simulink model "kr_billiards_exam"  (R2017b)
settings: Solver=VariableStepAuto  StartTime=0.0  StopTime=40  RelTol=1e-3  EnableMultiTasking=on
PreLoadFcn:
  | addpath('Bill_Tables_STEP')
  | addpath('Skins')
  | addpath('Utilities')
  | addpath('Kuka_KR10_R1100_STEP')
model workspace (MATLAB code in the model file):
  | den=1.613292710828678e+03;
  | st=0.004;
  | Damping=0.2;
  | 
  | % Length of brick solid
  | L = 20; % cm
  | % Width of brick solid
  | W = 2; % cm
  | % Height of brick solid
  | H = 2; % cm
  | % Density of brick solid
  | rho = 1000; % kg/m^3
undefined symbols (not defined in the file or in its folder): ball_col, ball_x, ball_y, X, Y, Z
libraries: sm_lib x83, nesl_utility x64, fl_lib x12, simulink x5
(part 1 of 4)
settings Model: Creator=User  LastModifiedBy=Boris S. Notkin
settings DataIOCC: LimitDataPoints=on  SaveOutput=off  SignalLogging=off  DSMLogging=off  SaveTime=off
settings OptimizationCC: LifeSpan=inf
settings DebuggingCC: AllowSymbolicDim=off  SFUnexpectedBacktrackingDiag=warning  SFNoUnconditionalDefaultTransitionDiag=warning  SFExecutionAtInitializationDiag=none
settings CodeAppCC: StateflowObjectComments=on
settings GRTTargetCC: TargetLangStandard=C89/C90 (ANSI)  GeneratePreprocessorConditionals=Disable all
settings ConfigComp: CovMetricSettings=dw  CovHtmlReporting=on  CovSaveCumulativeToWorkspaceVar=on  CovSaveSingleToWorkspaceVar=on  CovExternalEMLEnable=off  CovSFcnEnable=off
settings SimscapeCC: SimscapeNominalValues="[{\"value\":\"10\",\"unit\":\"V\"},{\"value\":\"1\",\"unit\":\"A\"},{\"value\":\"10\",\"unit\":\"N*m\"},{\"value\":\"10\",\"unit\":\"bar\"},{\"value\":\"100\",\"unit\":\"kJ/kg\"},{\"value\":\"1\",\"unit\":\"kW\"},{\"value\":\"300\",\"unit\":\"K\"},{\"value\":\"100\",\"unit\":\"cm^3/s\"},{\"value\":\"1\",\"unit\":\"kN\"},{\"value\":\"1\",\"unit\":\"g/cm^3\"},{\"value\":\"1\",\"unit\":\"l\"},{\"value\":\"1\",\"unit\":\"cm^2\"},{\"value\":\"60\",\"unit\":\"Hz\"}]"  SimscapeLogDataHistory=10000
settings ExplorerConfigSet: InternalSimMechanicsExplorerSettings="<ExplorerConfiguration><canonicalview>default</canonicalview><AnimationSetting><BasePlaybackSpeed>1.0</BasePlaybackSpeed><PlaybackSpeedFactor>1.0</PlaybackSpeedFactor></AnimationSetting><TilePanel><TileInfo><Tiles Columns=\"1\" Count=\"1\" Rows=\"1\"><Column Weight=\"1\"/><Row Weight=\"1\"/><Tile Height=\"1\" Width=\"1\" X=\"0\" Y=\"0\"/></Tiles></TileInfo><SceneInfo><SceneViewer><BGColor><R>0.60000002384185791</R><G>0.60000002384185791</G><B>0.60000002384185791</B></BGColor><Camera><DoPerspective>off</DoPerspective><Position><X>2.11392585240804332</X><Y>-1.25242729688440968</Y><Z>1.30776618684503054</Z></Position><Center><X>0.66802137799346617</X><Y>0.19347717753016791</Y><Z>-0.138138287569547241</Z></Center><Up><X>-0.408248290463863073</X><Y>0.408248290463863073</Y><Z>0.816496580927726145</Z></Up><ViewLimDist>1</ViewLimDist><YLim>0.89923064778922468</YLim><XLim>1.35470687907166232</XLim></Camera></SceneViewer></SceneInfo></TilePanel><MechEditorPanel><Cameras><Camera><Id>Camera1</Id><Value><Name>Robot Camera</Name><NativeCamera><PositionTrackingFeature>Kuka_KR10.Axis7_R</PositionTrackingFeature><CenterTrackingFeature/><UpVectorTrackingFeature/><CenterTrackingOrigin>off</CenterTrackingOrigin><CenterTrackingDirection>+Z</CenterTrackingDirection><UpVectorTrackingDirection>-X</UpVectorTrackingDirection></NativeCamera></Value></Camera></Cameras><GfxPanelCameraMap/><VideoCreator><PlaybackSpeedRatio>1.0</PlaybackSpeedRatio><FrameRate>30</FrameRate><VideoFormat>Motion JPEG AVI</VideoFormat><FrameSize>auto</FrameSize></VideoCreator></MechEditorPanel></ExplorerConfiguration>"

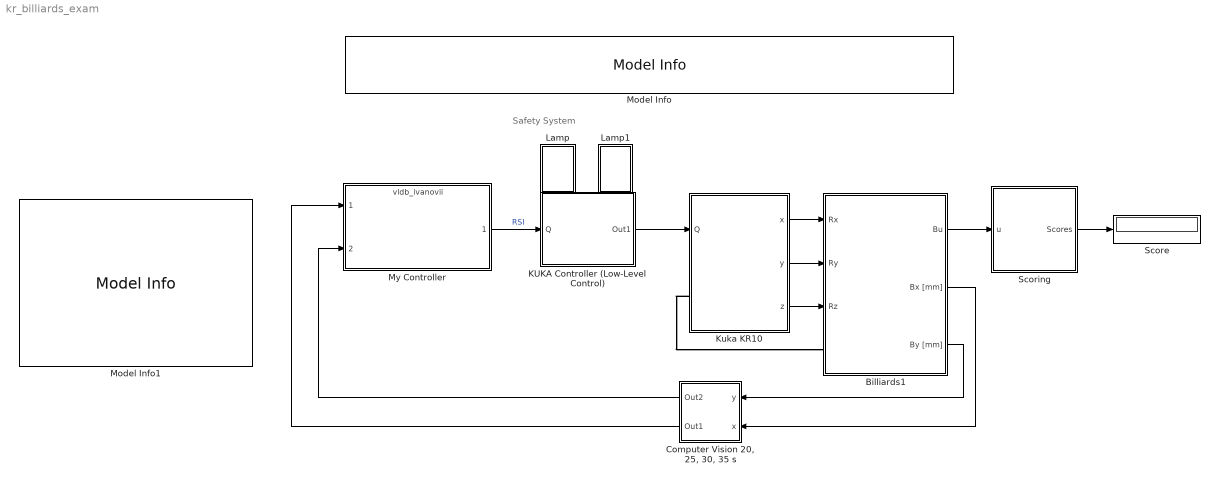
== system kr_billiards_exam ==
  note: Safety System
  Billiards1 : Subsystem
      mask init:
      | % [ball_x, ball_y, ball_col] = ball_and_cam_init_allocation(ball_mode, ball_rndfix, ...
      | %     ball_seed, foto_mode, foto_rndfix, foto_seed);
      mask DialogControl DescGroupVar Prompt: Размещение шаров на бильярдном столе и схема перемещения фотокамеры
      mask DialogControl DescTextVar Prompt: Выбор схемы размещения шаров на бильярдном шаре и схемы его обхода роботом, несущим фотокамеру системы компьютерного зрения.
      mask Display: image('billiard.jpg');
  "Computer Vision 20, 25, 30, 35 s" : Subsystem
      mask Display: image('comp_vis.jpg');
  KUKA Controller (Low-Level Control) : Subsystem  mask{min1=-170, max1=170, min2=-190, max2=45, min3=-120, max3=156, min4=-185, max4=185, min5=-120, max5=120, min6=-350, max6=350, EnableKinLim=on, acc1=600, acc2=450, acc3=450, acc4=762, acc5=622, acc6=984, EnableDynLim=on}
      mask prompts: min1 "Ось 1:"; min2 "Ось 2:"; min3 "Ось 3:"; min4 "Ось 4:"; min5 "Ось 5:"; min6 "Ось 6:"; EnableKinLim "Останавливать симуляцию при выходе за ограничения"; acc1 "Ось 1:"; acc2 "Ось 2:"; acc3 "Ось 3:"; acc4 "Ось 4:"; acc5 "Ось 5:"; acc6 "Ось 6:"; EnableDynLim "Останавливать симуляцию при выходе за ограничения"
      mask Callback EnableKinLim:
      | vis={'on','on','on','on','on','on','on','on','on','on','on','on','on','on','on','on','on','on','on','on'};
      | if strcmp(get_param(gcb,'EnableKinLim'),'off')
      |     for i=1:12
      |         vis{i}='off';
      |     end
      | end
      | if strcmp(get_param(gcb,'EnableDynLim'),'off')
      |     for i=14:19
      |         vis{i}='off';
      |     end
      | end
      | set_param(gcb,'MaskEnables',vis)
      mask Callback EnableDynLim:
      | vis={'on','on','on','on','on','on','on','on','on','on','on','on','on','on','on','on','on','on','on','on'};
      | if strcmp(get_param(gcb,'EnableKinLim'),'off')
      |     for i=1:12
      |         vis{i}='off';
      |     end
      | end
      | if strcmp(get_param(gcb,'EnableDynLim'),'off')
      |     for i=14:19
      |         vis{i}='off';
      |     end
      | end
      | set_param(gcb,'MaskEnables',vis)
      mask DialogControl ParameterGroupVar Prompt: Кинематические ограничения, град
      mask DialogControl Container3 Prompt: Динамические ограничения, град/c^2
      mask Display:
      | image('KR_C4.jpg');
      | port_label('input', 1, 'RSI')
  Kuka KR10 : Subsystem
      mask Display: image('kuka_kr10_r1100.jpg');
  Lamp : Subsystem  DialogController=hmiCreateDDGDialog  IsWebBlock=on  mask(MWDashboardBlock){webBlockId=50f85813-49c3-43b3-bc1d-ae04d07702bf, webBlockType=lamp, ShowInLibBrowser=on, ShowInitialText=on, HMISrcModelName=kr_billiards_exam}
      mask prompts: webBlockType "WebBlock Type"; HMISrcModelName "Source Model"
      mask help: SimulinkHMI:dialogs:LampDialogDesc
      mask Help: helpview([docroot '/mapfiles/simulink.map'], 'hmi_lamp')
      mask Display:
      | if strcmp(get_param(bdroot(gcb),'BlockDiagramType'), 'library')
      |     image([(matlabroot) '/toolbox/simulink/hmi/icons/Lamp.png']);
      | end
  Lamp1 : Subsystem  DialogController=hmiCreateDDGDialog  IsWebBlock=on  mask(MWDashboardBlock){webBlockId=c451b107-4d97-4e78-bf4d-8fc7e34e44b4, webBlockType=lamp, ShowInLibBrowser=on, ShowInitialText=on, HMISrcModelName=kr_billiards_exam}
      mask prompts: webBlockType "WebBlock Type"; HMISrcModelName "Source Model"
      mask help: SimulinkHMI:dialogs:LampDialogDesc
      mask Help: helpview([docroot '/mapfiles/simulink.map'], 'hmi_lamp')
      mask Display:
      | if strcmp(get_param(bdroot(gcb),'BlockDiagramType'), 'library')
      |     image([(matlabroot) '/toolbox/simulink/hmi/icons/Lamp.png']);
      | end
  Model Info : simulink/Model-Wide Utilities/Model Info  Frame=on  DisplayStringWithTags=Для запуска модели используйте скрипт EXAMINATOR.m  HorizontalTextAlignment=Center  LeftAlignmentValue=0.5
  Model Info1 : simulink/Model-Wide Utilities/Model Info  Frame=on  DisplayStringWithTags=|  HorizontalTextAlignment=Left  LeftAlignmentValue=0.02
      | Откройте на схеме блок My Controller (откроется 
      | модель участника) и в разделе описания модели
      | 
      | File/Model Properties//Model Properties/Description
      | 
      | укажите идентификационные данные участника 
      | Олимпиады.
      | 
      | 
      | Пример:
      | 
      | ФИО: Иванов Иван Иванович
      | ID: 123456789
      | Дата рождения: 23.02.1997
      | Email: ivanov@yandex.ru
      | Курс: Бакалавриат 4 курс
  My Controller : ModelReference  ModelNameDialog=vldb_ivanovii.slx  SimulationMode=Normal  ModelReferenceVersion=1.381
  Score : Display
  Scoring : Subsystem
      mask Display: image('scoring.jpg');
  wires:
  Kuka KR10/1(x) -> Billiards1/1(Rx)
  Kuka KR10/3(z) -> Billiards1/3(Rz)
  Kuka KR10/2(y) -> Billiards1/2(Ry)
  Billiards1/1(Bu) -> Scoring/1(u)
  Scoring/1(Scores) -> Score/1
  KUKA Controller (Low-Level Control)/1(Out1) -> Kuka KR10/1(Q)
  Billiards1/2(Bx [mm]) -> "Computer Vision 20, 25, 30, 35 s"/2(x)
  Billiards1/3(By [mm]) -> "Computer Vision 20, 25, 30, 35 s"/1(y)
  "Computer Vision 20, 25, 30, 35 s"/1(Out2) -> My Controller/2
  "Computer Vision 20, 25, 30, 35 s"/2(Out1) -> My Controller/1
  My Controller/1 -> KUKA Controller (Low-Level Control)/1(Q)  "RSI"
  connections:
  Kuka KR10/LConn1 -- Billiards1/LConn1

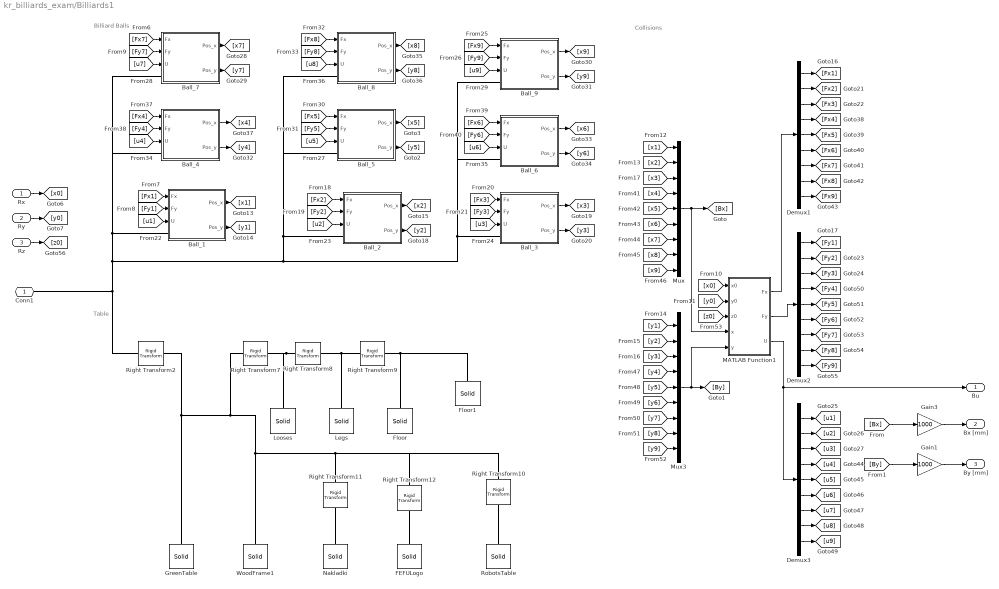
== system kr_billiards_exam/Billiards1 ==
  note: Collisions
  note: Billiard Balls
  note: Table
  Rx : Inport
  Ry : Inport  Port=2
  Rz : Inport  Port=3
  Ball_1 : Subsystem  mask{x0=ball_x(1), y0=ball_y(1), d=Damping, pd=5, rgb=ball_col(1,:)}
      mask prompts: d "Damping"; pd "Parking damping"; rgb "Color"
  Ball_2 : Subsystem  mask{x0=ball_x(2), y0=ball_y(2), d=Damping, pd=5, rgb=ball_col(2,:)}
      mask prompts: d "Damping"; pd "Parking damping"; rgb "Color"
  Ball_3 : Subsystem  mask{x0=ball_x(3), y0=ball_y(3), d=Damping, pd=5, rgb=ball_col(3,:)}
      mask prompts: d "Damping"; pd "Parking damping"; rgb "Color"
  Ball_4 : Subsystem  mask{x0=ball_x(4), y0=ball_y(4), d=Damping, pd=5, rgb=ball_col(4,:)}
      mask prompts: d "Damping"; pd "Parking damping"; rgb "Color"
  Ball_5 : Subsystem  mask{x0=ball_x(5), y0=ball_y(5), d=Damping, pd=5, rgb=ball_col(5,:)}
      mask prompts: d "Damping"; pd "Parking damping"; rgb "Color"
  Ball_6 : Subsystem  mask{x0=ball_x(6), y0=ball_y(6), d=Damping, pd=5, rgb=ball_col(6,:)}
      mask prompts: d "Damping"; pd "Parking damping"; rgb "Color"
  Ball_7 : Subsystem  mask{x0=ball_x(7), y0=ball_y(7), d=Damping, pd=5, rgb=ball_col(7,:)}
      mask prompts: d "Damping"; pd "Parking damping"; rgb "Color"
  Ball_8 : Subsystem  mask{x0=ball_x(8), y0=ball_y(8), d=Damping, pd=5, rgb=ball_col(8,:)}
      mask prompts: d "Damping"; pd "Parking damping"; rgb "Color"
  Ball_9 : Subsystem  mask{x0=ball_x(9), y0=ball_y(9), d=Damping, pd=5, rgb=ball_col(9,:)}
      mask prompts: d "Damping"; pd "Parking damping"; rgb "Color"
  Demux1 : Demux  Outputs=9
  Demux2 : Demux  Outputs=9
  Demux3 : Demux  Outputs=9
  FEFULogo : sm_lib/Body Elements/Solid  InertiaType=CalculateFromGeometry  Mass=1  MassUnits=kg  CenterOfMass=[0 0 0]  CenterOfMassUnits=m  MomentsOfInertia=[1 1 1]  MomentsOfInertiaUnits=kg*m^2  ProductsOfInertia=[0 0 0]  ProductsOfInertiaUnits=kg*m^2  DensityBased=on  Density=rho  DensityUnits=kg/m^3  DoExposeReferenceFrame=on  SerializedFrames=<Frames/>  GraphicType=FromGeometry  MarkerShape=Sphere  MarkerSize=1  MarkerSizeUnits=m  GraphicVisPropType=SimpleVisualProperties  GraphicDiffuseColor=[1.0 0.8 0.0]  GraphicSpecularColor=[0.2 0.2 0.2]  GraphicAmbientColor=[0.5 0.5 0.5]  GraphicEmissiveColor=[0.1 0.1 0.1]  GraphicShininess=24.0  GraphicOpacity=1  GeometryShape=FromFile  RectangleSize=[1 1]  RectangleSizeUnits=m  BrickDimensions=[L W H]  BrickDimensionUnits=cm  CylinderRadius=1  CylinderRadiusUnits=m  CylinderLength=1  CylinderLengthUnits=m  SphereRadius=1  SphereRadiusUnits=m  EllipsoidRadii=[1 1 1]  EllipsoidRadiiUnits=m  ExtrusionCrossSection=[1 1; -1 1; -1 -1; 1 -1]  ExtrusionCrossSectionUnits=m  ExtrusionLength=1  ExtrusionLengthUnits=m  PolygonNumSides=1  PolygonOuterRadius=1  PolygonOuterRadiusUnits=m  ExtGeomFileType=STEP  ExtGeomFileName=FEFULogo.STEP  ExtGeomFileUnits=m  RevolutionCrossSection=[1 1; 1 -1; 2 -1; 2 1]  RevolutionCrossSectionUnits=m  RevolutionExtent=Full  RevolutionAngle=180  RevolutionAngleUnits=deg
  Floor : sm_lib/Body Elements/Solid  InertiaType=CalculateFromGeometry  Mass=1  MassUnits=kg  CenterOfMass=[0 0 0]  CenterOfMassUnits=m  MomentsOfInertia=[1 1 1]  MomentsOfInertiaUnits=kg*m^2  ProductsOfInertia=[0 0 0]  ProductsOfInertiaUnits=kg*m^2  DensityBased=on  Density=rho  DensityUnits=kg/m^3  DoExposeReferenceFrame=on  SerializedFrames=<Frames/>  GraphicType=FromGeometry  MarkerShape=Sphere  MarkerSize=1  MarkerSizeUnits=m  GraphicVisPropType=SimpleVisualProperties  GraphicDiffuseColor=[1.0 1.0 1.0]  GraphicSpecularColor=[0.2 0.2 0.2]  GraphicAmbientColor=[0.5 0.5 0.5]  GraphicEmissiveColor=[0.1 0.1 0.1]  GraphicShininess=24.0  GraphicOpacity=1  GeometryShape=FromFile  RectangleSize=[1 1]  RectangleSizeUnits=m  BrickDimensions=[L W H]  BrickDimensionUnits=cm  CylinderRadius=1  CylinderRadiusUnits=m  CylinderLength=1  CylinderLengthUnits=m  SphereRadius=1  SphereRadiusUnits=m  EllipsoidRadii=[1 1 1]  EllipsoidRadiiUnits=m  ExtrusionCrossSection=[1 1; -1 1; -1 -1; 1 -1]  ExtrusionCrossSectionUnits=m  ExtrusionLength=1  ExtrusionLengthUnits=m  PolygonNumSides=1  PolygonOuterRadius=1  PolygonOuterRadiusUnits=m  ExtGeomFileType=STEP  ExtGeomFileName=Floor.STEP  ExtGeomFileUnits=m  RevolutionCrossSection=[1 1; 1 -1; 2 -1; 2 1]  RevolutionCrossSectionUnits=m  RevolutionExtent=Full  RevolutionAngle=180  RevolutionAngleUnits=deg
  Floor1 : sm_lib/Body Elements/Solid  InertiaType=CalculateFromGeometry  Mass=1  MassUnits=kg  CenterOfMass=[0 0 0]  CenterOfMassUnits=m  MomentsOfInertia=[1 1 1]  MomentsOfInertiaUnits=kg*m^2  ProductsOfInertia=[0 0 0]  ProductsOfInertiaUnits=kg*m^2  DensityBased=on  Density=rho  DensityUnits=kg/m^3  DoExposeReferenceFrame=on  SerializedFrames=<Frames/>  GraphicType=FromGeometry  MarkerShape=Sphere  MarkerSize=1  MarkerSizeUnits=m  GraphicVisPropType=SimpleVisualProperties  GraphicDiffuseColor=[0.3 0.3 0.3]  GraphicSpecularColor=[0.2 0.2 0.2]  GraphicAmbientColor=[0.5 0.5 0.5]  GraphicEmissiveColor=[0.1 0.1 0.1]  GraphicShininess=24.0  GraphicOpacity=1  GeometryShape=Brick  RectangleSize=[1 1]  RectangleSizeUnits=m  BrickDimensions=[6 3 0.003]  BrickDimensionUnits=m  CylinderRadius=1  CylinderRadiusUnits=m  CylinderLength=1  CylinderLengthUnits=m  SphereRadius=1  SphereRadiusUnits=m  EllipsoidRadii=[1 1 1]  EllipsoidRadiiUnits=m  ExtrusionCrossSection=[1 1; -1 1; -1 -1; 1 -1]  ExtrusionCrossSectionUnits=m  ExtrusionLength=1  ExtrusionLengthUnits=m  PolygonNumSides=1  PolygonOuterRadius=1  PolygonOuterRadiusUnits=m  ExtGeomFileType=STEP  ExtGeomFileName=C:\PingPong\BillTablesSTEPDecor2\Floor.STEP  ExtGeomFileUnits=m  RevolutionCrossSection=[1 1; 1 -1; 2 -1; 2 1]  RevolutionCrossSectionUnits=m  RevolutionExtent=Full  RevolutionAngle=180  RevolutionAngleUnits=deg
  Gain1 : Gain  Gain=1000
  Gain3 : Gain  Gain=1000
  GreenTable : sm_lib/Body Elements/Solid  InertiaType=CalculateFromGeometry  Mass=1  MassUnits=kg  CenterOfMass=[0 0 0]  CenterOfMassUnits=m  MomentsOfInertia=[1 1 1]  MomentsOfInertiaUnits=kg*m^2  ProductsOfInertia=[0 0 0]  ProductsOfInertiaUnits=kg*m^2  DensityBased=on  Density=rho  DensityUnits=kg/m^3  DoExposeReferenceFrame=on  SerializedFrames=<Frames/>  GraphicType=FromGeometry  MarkerShape=Sphere  MarkerSize=1  MarkerSizeUnits=m  GraphicVisPropType=SimpleVisualProperties  GraphicDiffuseColor=[0.0 0.8 0.2]  GraphicSpecularColor=[0.2 0.2 0.2]  GraphicAmbientColor=[0.5 0.5 0.5]  GraphicEmissiveColor=[0.1 0.1 0.1]  GraphicShininess=24.0  GraphicOpacity=1  GeometryShape=FromFile  RectangleSize=[1 1]  RectangleSizeUnits=m  BrickDimensions=[L W H]  BrickDimensionUnits=cm  CylinderRadius=1  CylinderRadiusUnits=m  CylinderLength=1  CylinderLengthUnits=m  SphereRadius=1  SphereRadiusUnits=m  EllipsoidRadii=[1 1 1]  EllipsoidRadiiUnits=m  ExtrusionCrossSection=[1 1; -1 1; -1 -1; 1 -1]  ExtrusionCrossSectionUnits=m  ExtrusionLength=1  ExtrusionLengthUnits=m  PolygonNumSides=1  PolygonOuterRadius=1  PolygonOuterRadiusUnits=m  ExtGeomFileType=STEP  ExtGeomFileName=GreenTable.STEP  ExtGeomFileUnits=m  RevolutionCrossSection=[1 1; 1 -1; 2 -1; 2 1]  RevolutionCrossSectionUnits=m  RevolutionExtent=Full  RevolutionAngle=180  RevolutionAngleUnits=deg
  Legs : sm_lib/Body Elements/Solid  InertiaType=CalculateFromGeometry  Mass=1  MassUnits=kg  CenterOfMass=[0 0 0]  CenterOfMassUnits=m  MomentsOfInertia=[1 1 1]  MomentsOfInertiaUnits=kg*m^2  ProductsOfInertia=[0 0 0]  ProductsOfInertiaUnits=kg*m^2  DensityBased=on  Density=rho  DensityUnits=kg/m^3  DoExposeReferenceFrame=on  SerializedFrames=<Frames/>  GraphicType=FromGeometry  MarkerShape=Sphere  MarkerSize=1  MarkerSizeUnits=m  GraphicVisPropType=SimpleVisualProperties  GraphicDiffuseColor=[1.0 0.8 0.4]  GraphicSpecularColor=[0.2 0.2 0.2]  GraphicAmbientColor=[0.5 0.5 0.5]  GraphicEmissiveColor=[0.1 0.1 0.1]  GraphicShininess=24.0  GraphicOpacity=1  GeometryShape=FromFile  RectangleSize=[1 1]  RectangleSizeUnits=m  BrickDimensions=[L W H]  BrickDimensionUnits=cm  CylinderRadius=1  CylinderRadiusUnits=m  CylinderLength=1  CylinderLengthUnits=m  SphereRadius=1  SphereRadiusUnits=m  EllipsoidRadii=[1 1 1]  EllipsoidRadiiUnits=m  ExtrusionCrossSection=[1 1; -1 1; -1 -1; 1 -1]  ExtrusionCrossSectionUnits=m  ExtrusionLength=1  ExtrusionLengthUnits=m  PolygonNumSides=1  PolygonOuterRadius=1  PolygonOuterRadiusUnits=m  ExtGeomFileType=STEP  ExtGeomFileName=Legs.STEP  ExtGeomFileUnits=m  RevolutionCrossSection=[1 1; 1 -1; 2 -1; 2 1]  RevolutionCrossSectionUnits=m  RevolutionExtent=Full  RevolutionAngle=180  RevolutionAngleUnits=deg
  Looses : sm_lib/Body Elements/Solid  InertiaType=CalculateFromGeometry  Mass=1  MassUnits=kg  CenterOfMass=[0 0 0]  CenterOfMassUnits=m  MomentsOfInertia=[1 1 1]  MomentsOfInertiaUnits=kg*m^2  ProductsOfInertia=[0 0 0]  ProductsOfInertiaUnits=kg*m^2  DensityBased=on  Density=rho  DensityUnits=kg/m^3  DoExposeReferenceFrame=on  SerializedFrames=<Frames/>  GraphicType=FromGeometry  MarkerShape=Sphere  MarkerSize=1  MarkerSizeUnits=m  GraphicVisPropType=SimpleVisualProperties  GraphicDiffuseColor=[0.2 0.2 0.2]  GraphicSpecularColor=[0.2 0.2 0.2]  GraphicAmbientColor=[0.5 0.5 0.5]  GraphicEmissiveColor=[0.1 0.1 0.1]  GraphicShininess=24.0  GraphicOpacity=1  GeometryShape=FromFile  RectangleSize=[1 1]  RectangleSizeUnits=m  BrickDimensions=[L W H]  BrickDimensionUnits=cm  CylinderRadius=1  CylinderRadiusUnits=m  CylinderLength=1  CylinderLengthUnits=m  SphereRadius=1  SphereRadiusUnits=m  EllipsoidRadii=[1 1 1]  EllipsoidRadiiUnits=m  ExtrusionCrossSection=[1 1; -1 1; -1 -1; 1 -1]  ExtrusionCrossSectionUnits=m  ExtrusionLength=1  ExtrusionLengthUnits=m  PolygonNumSides=1  PolygonOuterRadius=1  PolygonOuterRadiusUnits=m  ExtGeomFileType=STEP  ExtGeomFileName=Looses.STEP  ExtGeomFileUnits=m  RevolutionCrossSection=[1 1; 1 -1; 2 -1; 2 1]  RevolutionCrossSectionUnits=m  RevolutionExtent=Full  RevolutionAngle=180  RevolutionAngleUnits=deg
  MATLAB Function1 : MATLAB Function  TreatAsAtomicUnit=on
  Mux : Mux  Inputs=9
  Mux3 : Mux  Inputs=9
  Nakladki : sm_lib/Body Elements/Solid  InertiaType=CalculateFromGeometry  Mass=1  MassUnits=kg  CenterOfMass=[0 0 0]  CenterOfMassUnits=m  MomentsOfInertia=[1 1 1]  MomentsOfInertiaUnits=kg*m^2  ProductsOfInertia=[0 0 0]  ProductsOfInertiaUnits=kg*m^2  DensityBased=on  Density=rho  DensityUnits=kg/m^3  DoExposeReferenceFrame=on  SerializedFrames=<Frames/>  GraphicType=FromGeometry  MarkerShape=Sphere  MarkerSize=1  MarkerSizeUnits=m  GraphicVisPropType=SimpleVisualProperties  GraphicDiffuseColor=[1.0 0.8 0.0]  GraphicSpecularColor=[0.2 0.2 0.2]  GraphicAmbientColor=[0.5 0.5 0.5]  GraphicEmissiveColor=[0.1 0.1 0.1]  GraphicShininess=24.0  GraphicOpacity=1  GeometryShape=FromFile  RectangleSize=[1 1]  RectangleSizeUnits=m  BrickDimensions=[L W H]  BrickDimensionUnits=cm  CylinderRadius=1  CylinderRadiusUnits=m  CylinderLength=1  CylinderLengthUnits=m  SphereRadius=1  SphereRadiusUnits=m  EllipsoidRadii=[1 1 1]  EllipsoidRadiiUnits=m  ExtrusionCrossSection=[1 1; -1 1; -1 -1; 1 -1]  ExtrusionCrossSectionUnits=m  ExtrusionLength=1  ExtrusionLengthUnits=m  PolygonNumSides=1  PolygonOuterRadius=1  PolygonOuterRadiusUnits=m  ExtGeomFileType=STEP  ExtGeomFileName=Nakladki.STEP  ExtGeomFileUnits=m  RevolutionCrossSection=[1 1; 1 -1; 2 -1; 2 1]  RevolutionCrossSectionUnits=m  RevolutionExtent=Full  RevolutionAngle=180  RevolutionAngleUnits=deg
  Right Transform10 : sm_lib/Frames and Transforms/Rigid Transform  TranslationMethod=Cartesian  TranslationStandardOffset=L/2  TranslationLengthUnit=mm  TranslationStandardAxis=+X  TranslationCartesianOffset=[0 0 -523.67]  TranslationROffset=0  TranslationROffsetUnits=m  TranslationZOffset=0  TranslationZOffsetUnits=m  TranslationThetaOffset=0  TranslationThetaOffsetUnits=deg  RotationMethod=AlignedAxes  RotationAngleUnits=deg  RotationStandardAxis=+Z  RotationAngle=0  RotationArbitraryAxis=[0 0 1]  FollAlignAxisA=+Z  BaseAlignAxisA=+Z  FollAlignAxisB=+X  BaseAlignAxisB=+X  RotationSequenceAxes=FollowerAxes  RotationSequence=XYX  RotationSequenceAngles=[0 0 0]  RotationSequenceAnglesUnits=deg  RotationMatrix=[1 0 0; 0 1 0; 0 0 1]
  Right Transform11 : sm_lib/Frames and Transforms/Rigid Transform  TranslationMethod=Cartesian  TranslationStandardOffset=L/2  TranslationLengthUnit=mm  TranslationStandardAxis=+X  TranslationCartesianOffset=[0 50 0]  TranslationROffset=0  TranslationROffsetUnits=m  TranslationZOffset=0  TranslationZOffsetUnits=m  TranslationThetaOffset=0  TranslationThetaOffsetUnits=deg  RotationMethod=AlignedAxes  RotationAngleUnits=deg  RotationStandardAxis=+Z  RotationAngle=0  RotationArbitraryAxis=[0 0 1]  FollAlignAxisA=+Z  BaseAlignAxisA=+Y  FollAlignAxisB=+Y  BaseAlignAxisB=+Z  RotationSequenceAxes=FollowerAxes  RotationSequence=XYX  RotationSequenceAngles=[0 0 0]  RotationSequenceAnglesUnits=deg  RotationMatrix=[1 0 0; 0 1 0; 0 0 1]
  Right Transform12 : sm_lib/Frames and Transforms/Rigid Transform  TranslationMethod=Cartesian  TranslationStandardOffset=L/2  TranslationLengthUnit=mm  TranslationStandardAxis=+X  TranslationCartesianOffset=[0 -460.09 0]  TranslationROffset=0  TranslationROffsetUnits=m  TranslationZOffset=0  TranslationZOffsetUnits=m  TranslationThetaOffset=0  TranslationThetaOffsetUnits=deg  RotationMethod=AlignedAxes  RotationAngleUnits=deg  RotationStandardAxis=+Z  RotationAngle=0  RotationArbitraryAxis=[0 0 1]  FollAlignAxisA=+Z  BaseAlignAxisA=+Z  FollAlignAxisB=+X  BaseAlignAxisB=+X  RotationSequenceAxes=FollowerAxes  RotationSequence=XYX  RotationSequenceAngles=[0 0 0]  RotationSequenceAnglesUnits=deg  RotationMatrix=[1 0 0; 0 1 0; 0 0 1]
  Right Transform2 : sm_lib/Frames and Transforms/Rigid Transform  TranslationMethod=Cartesian  TranslationStandardOffset=L/2  TranslationLengthUnit=mm  TranslationStandardAxis=+X  TranslationCartesianOffset=[725 0 70]  TranslationROffset=0  TranslationROffsetUnits=m  TranslationZOffset=0  TranslationZOffsetUnits=m  TranslationThetaOffset=0  TranslationThetaOffsetUnits=deg  RotationMethod=RotationSequence  RotationAngleUnits=deg  RotationStandardAxis=+Z  RotationAngle=0  RotationArbitraryAxis=[0 0 1]  FollAlignAxisA=+X  BaseAlignAxisA=-Y  FollAlignAxisB=+Y  BaseAlignAxisB=-X  RotationSequenceAxes=FollowerAxes  RotationSequence=ZYX  RotationSequenceAngles=[90 0 90]  RotationSequenceAnglesUnits=deg  RotationMatrix=[1 0 0; 0 1 0; 0 0 1]
  Right Transform7 : sm_lib/Frames and Transforms/Rigid Transform  TranslationMethod=Cartesian  TranslationStandardOffset=L/2  TranslationLengthUnit=mm  TranslationStandardAxis=+X  TranslationCartesianOffset=[0 0 0]  TranslationROffset=0  TranslationROffsetUnits=m  TranslationZOffset=0  TranslationZOffsetUnits=m  TranslationThetaOffset=0  TranslationThetaOffsetUnits=deg  RotationMethod=AlignedAxes  RotationAngleUnits=deg  RotationStandardAxis=+Z  RotationAngle=0  RotationArbitraryAxis=[0 0 1]  FollAlignAxisA=+Z  BaseAlignAxisA=+Y  FollAlignAxisB=+Y  BaseAlignAxisB=+Z  RotationSequenceAxes=FollowerAxes  RotationSequence=XYX  RotationSequenceAngles=[0 0 0]  RotationSequenceAnglesUnits=deg  RotationMatrix=[1 0 0; 0 1 0; 0 0 1]
  Right Transform8 : sm_lib/Frames and Transforms/Rigid Transform  TranslationMethod=Cartesian  TranslationStandardOffset=L/2  TranslationLengthUnit=mm  TranslationStandardAxis=+X  TranslationCartesianOffset=[0 0 0]  TranslationROffset=0  TranslationROffsetUnits=m  TranslationZOffset=0  TranslationZOffsetUnits=m  TranslationThetaOffset=0  TranslationThetaOffsetUnits=deg  RotationMethod=AlignedAxes  RotationAngleUnits=deg  RotationStandardAxis=+Z  RotationAngle=0  RotationArbitraryAxis=[0 0 1]  FollAlignAxisA=+Z  BaseAlignAxisA=+Y  FollAlignAxisB=+Y  BaseAlignAxisB=+Z  RotationSequenceAxes=FollowerAxes  RotationSequence=XYX  RotationSequenceAngles=[0 0 0]  RotationSequenceAnglesUnits=deg  RotationMatrix=[1 0 0; 0 1 0; 0 0 1]
  Right Transform9 : sm_lib/Frames and Transforms/Rigid Transform  TranslationMethod=Cartesian  TranslationStandardOffset=L/2  TranslationLengthUnit=mm  TranslationStandardAxis=+X  TranslationCartesianOffset=[0 -461.09 0]  TranslationROffset=0  TranslationROffsetUnits=m  TranslationZOffset=0  TranslationZOffsetUnits=m  TranslationThetaOffset=0  TranslationThetaOffsetUnits=deg  RotationMethod=AlignedAxes  RotationAngleUnits=deg  RotationStandardAxis=+Z  RotationAngle=0  RotationArbitraryAxis=[0 0 1]  FollAlignAxisA=+Z  BaseAlignAxisA=+Y  FollAlignAxisB=+Y  BaseAlignAxisB=+Z  RotationSequenceAxes=FollowerAxes  RotationSequence=XYX  RotationSequenceAngles=[0 0 0]  RotationSequenceAnglesUnits=deg  RotationMatrix=[1 0 0; 0 1 0; 0 0 1]
  RobotsTable : sm_lib/Body Elements/Solid  InertiaType=CalculateFromGeometry  Mass=1  MassUnits=kg  CenterOfMass=[0 0 0]  CenterOfMassUnits=m  MomentsOfInertia=[1 1 1]  MomentsOfInertiaUnits=kg*m^2  ProductsOfInertia=[0 0 0]  ProductsOfInertiaUnits=kg*m^2  DensityBased=on  Density=rho  DensityUnits=kg/m^3  DoExposeReferenceFrame=on  SerializedFrames=<Frames/>  GraphicType=FromGeometry  MarkerShape=Sphere  MarkerSize=1  MarkerSizeUnits=m  GraphicVisPropType=SimpleVisualProperties  GraphicDiffuseColor=[0.4 0.4 0.4]  GraphicSpecularColor=[0.2 0.2 0.2]  GraphicAmbientColor=[0.5 0.5 0.5]  GraphicEmissiveColor=[0.1 0.1 0.1]  GraphicShininess=24.0  GraphicOpacity=1  GeometryShape=FromFile  RectangleSize=[1 1]  RectangleSizeUnits=m  BrickDimensions=[L W H]  BrickDimensionUnits=cm  CylinderRadius=1  CylinderRadiusUnits=m  CylinderLength=1  CylinderLengthUnits=m  SphereRadius=1  SphereRadiusUnits=m  EllipsoidRadii=[1 1 1]  EllipsoidRadiiUnits=m  ExtrusionCrossSection=[1 1; -1 1; -1 -1; 1 -1]  ExtrusionCrossSectionUnits=m  ExtrusionLength=1  ExtrusionLengthUnits=m  PolygonNumSides=1  PolygonOuterRadius=1  PolygonOuterRadiusUnits=m  ExtGeomFileType=STEP  ExtGeomFileName=RobotsTable.STEP  ExtGeomFileUnits=m  RevolutionCrossSection=[1 1; 1 -1; 2 -1; 2 1]  RevolutionCrossSectionUnits=m  RevolutionExtent=Full  RevolutionAngle=180  RevolutionAngleUnits=deg
  WoodFrame1 : sm_lib/Body Elements/Solid  InertiaType=CalculateFromGeometry  Mass=1  MassUnits=kg  CenterOfMass=[0 0 0]  CenterOfMassUnits=m  MomentsOfInertia=[1 1 1]  MomentsOfInertiaUnits=kg*m^2  ProductsOfInertia=[0 0 0]  ProductsOfInertiaUnits=kg*m^2  DensityBased=on  Density=rho  DensityUnits=kg/m^3  DoExposeReferenceFrame=on  SerializedFrames=<Frames/>  GraphicType=FromGeometry  MarkerShape=Sphere  MarkerSize=1  MarkerSizeUnits=m  GraphicVisPropType=SimpleVisualProperties  GraphicDiffuseColor=[1.0 0.4 0.0]  GraphicSpecularColor=[0.2 0.2 0.2]  GraphicAmbientColor=[0.5 0.5 0.5]  GraphicEmissiveColor=[0.1 0.1 0.1]  GraphicShininess=24.0  GraphicOpacity=1  GeometryShape=FromFile  RectangleSize=[1 1]  RectangleSizeUnits=m  BrickDimensions=[L W H]  BrickDimensionUnits=cm  CylinderRadius=1  CylinderRadiusUnits=m  CylinderLength=1  CylinderLengthUnits=m  SphereRadius=1  SphereRadiusUnits=m  EllipsoidRadii=[1 1 1]  EllipsoidRadiiUnits=m  ExtrusionCrossSection=[1 1; -1 1; -1 -1; 1 -1]  ExtrusionCrossSectionUnits=m  ExtrusionLength=1  ExtrusionLengthUnits=m  PolygonNumSides=1  PolygonOuterRadius=1  PolygonOuterRadiusUnits=m  ExtGeomFileType=STEP  ExtGeomFileName=WoodFrame.STEP  ExtGeomFileUnits=m  RevolutionCrossSection=[1 1; 1 -1; 2 -1; 2 1]  RevolutionCrossSectionUnits=m  RevolutionExtent=Full  RevolutionAngle=180  RevolutionAngleUnits=deg
  Conn1 : PMIOPort  Port=1  Side=Left
  Bu : Outport
  Bx [mm] : Outport  Port=2
  By [mm] : Outport  Port=3
  wires:
  [u5] -> Ball_5/3(U)
  Ball_9/2(Pos_y) -> [y9]
  [Fy4] -> Ball_4/2(Fy)
  [u7] -> Ball_7/3(U)
  [Fy8] -> Ball_8/2(Fy)
  [Fx8] -> Ball_8/1(Fx)
  [Fy3] -> Ball_3/2(Fy)
  Ball_8/2(Pos_y) -> [y8]
  [Fy6] -> Ball_6/2(Fy)
  [Fy2] -> Ball_2/2(Fy)
  [Fx4] -> Ball_4/1(Fx)
  Ball_1/2(Pos_y) -> [y1]
  Ball_1/1(Pos_x) -> [x1]
  [u2] -> Ball_2/3(U)
  Ball_5/1(Pos_x) -> [x5]
  [u4] -> Ball_4/3(U)
  [Fx3] -> Ball_3/1(Fx)
  [Fy9] -> Ball_9/2(Fy)
  Ball_5/2(Pos_y) -> [y5]
  Ball_2/2(Pos_y) -> [y2]
  Ball_9/1(Pos_x) -> [x9]
  Ball_4/1(Pos_x) -> [x4]
  Ball_3/1(Pos_x) -> [x3]
  [u6] -> Ball_6/3(U)
  Ball_2/1(Pos_x) -> [x2]
  Ball_8/1(Pos_x) -> [x8]
  [Fx1] -> Ball_1/1(Fx)
  Ball_6/1(Pos_x) -> [x6]
  Ball_3/2(Pos_y) -> [y3]
  [u1] -> Ball_1/3(U)
  [Fx6] -> Ball_6/1(Fx)
  [Fy1] -> Ball_1/2(Fy)
  [Fy7] -> Ball_7/2(Fy)
  [u9] -> Ball_9/3(U)
  [Fx2] -> Ball_2/1(Fx)
  [Fx5] -> Ball_5/1(Fx)
  Ball_6/2(Pos_y) -> [y6]
  Ball_7/1(Pos_x) -> [x7]
  Ball_4/2(Pos_y) -> [y4]
  [Fx9] -> Ball_9/1(Fx)
  [u3] -> Ball_3/3(U)
  [Fx7] -> Ball_7/1(Fx)
  Ball_7/2(Pos_y) -> [y7]
  [u8] -> Ball_8/3(U)
  [Fy5] -> Ball_5/2(Fy)
  Rz/1 -> [z0]
  Rx/1 -> [x0]
  Ry/1 -> [y0]
  MATLAB Function1/1(Fx) -> Demux1/1
  Mux/1 -> [Bx], MATLAB Function1/4(x)
  Mux3/1 -> [By], MATLAB Function1/5(y)
  MATLAB Function1/3(U) -> Demux3/1, Bu/1
  MATLAB Function1/2(Fy) -> Demux2/1
  [z0] -> MATLAB Function1/3(z0)
  [x0] -> MATLAB Function1/1(x0)
  [y0] -> MATLAB Function1/2(y0)
  [x1] -> Mux/1
  [x2] -> Mux/2
  [x3] -> Mux/3
  [x4] -> Mux/4
  [x5] -> Mux/5
  [x6] -> Mux/6
  [x7] -> Mux/7
  [x8] -> Mux/8
  [x9] -> Mux/9
  [y1] -> Mux3/1
  [y2] -> Mux3/2
  [y3] -> Mux3/3
  [y4] -> Mux3/4
  [y5] -> Mux3/5
  [y6] -> Mux3/6
  [y7] -> Mux3/7
  [y8] -> Mux3/8
  [y9] -> Mux3/9
  Demux1/1 -> [Fx1]
  Demux1/2 -> [Fx2]
  Demux1/3 -> [Fx3]
  Demux1/4 -> [Fx4]
  Demux1/5 -> [Fx5]
  Demux1/6 -> [Fx6]
  Demux1/7 -> [Fx7]
  Demux1/8 -> [Fx8]
  Demux1/9 -> [Fx9]
  Demux2/1 -> [Fy1]
  Demux2/2 -> [Fy2]
  Demux2/3 -> [Fy3]
  Demux2/4 -> [Fy4]
  Demux2/5 -> [Fy5]
  Demux2/6 -> [Fy6]
  Demux2/7 -> [Fy7]
  Demux2/8 -> [Fy8]
  Demux2/9 -> [Fy9]
  Demux3/1 -> [u1]
  Demux3/2 -> [u2]
  Demux3/3 -> [u3]
  Demux3/4 -> [u4]
  Demux3/5 -> [u5]
  Demux3/6 -> [u6]
  Demux3/7 -> [u7]
  Demux3/8 -> [u8]
  Demux3/9 -> [u9]
  [Bx] -> Gain3/1
  [By] -> Gain1/1
  Gain3/1 -> Bx [mm]/1
  Gain1/1 -> By [mm]/1
  connections:
  Conn1/RConn1 -- Ball_7/LConn1 -- Ball_4/LConn1 -- Ball_1/LConn1 -- Ball_8/LConn1 -- Ball_5/LConn1 -- Ball_2/LConn1 -- Ball_9/LConn1 -- Ball_6/LConn1 -- Ball_3/LConn1 -- Right Transform2/LConn1
  Right Transform8/LConn1 -- Looses/RConn1 -- Right Transform7/RConn1
  Right Transform9/RConn1 -- Floor1/RConn1 -- Floor/RConn1
  Right Transform2/RConn1 -- GreenTable/RConn1 -- Right Transform10/LConn1 -- Right Transform12/LConn1 -- Right Transform11/LConn1 -- WoodFrame1/RConn1 -- Right Transform7/LConn1
  Legs/RConn1 -- Right Transform9/LConn1 -- Right Transform8/RConn1
  FEFULogo/RConn1 -- Right Transform12/RConn1
  Nakladki/RConn1 -- Right Transform11/RConn1
  Right Transform10/RConn1 -- RobotsTable/RConn1

== system kr_billiards_exam/Computer Vision 20, 25, 30, 35 s ==
  y : Inport
  x : Inport  Port=2
  Product : Product
  Product1 : Product
  Step1 : Step  Time=20  SampleTime=0
  Zero-Order Hold : ZeroOrderHold  SampleTime=5
  Zero-Order Hold1 : ZeroOrderHold  SampleTime=5
  Out2 : Outport
  Out1 : Outport  Port=2
  wires:
  Zero-Order Hold1/1 -> Product1/2
  Product/1 -> Out2/1
  Product1/1 -> Out1/1
  Zero-Order Hold/1 -> Product/2
  y/1 -> Zero-Order Hold/1
  x/1 -> Zero-Order Hold1/1
  Step1/1 -> Product1/1, Product/1

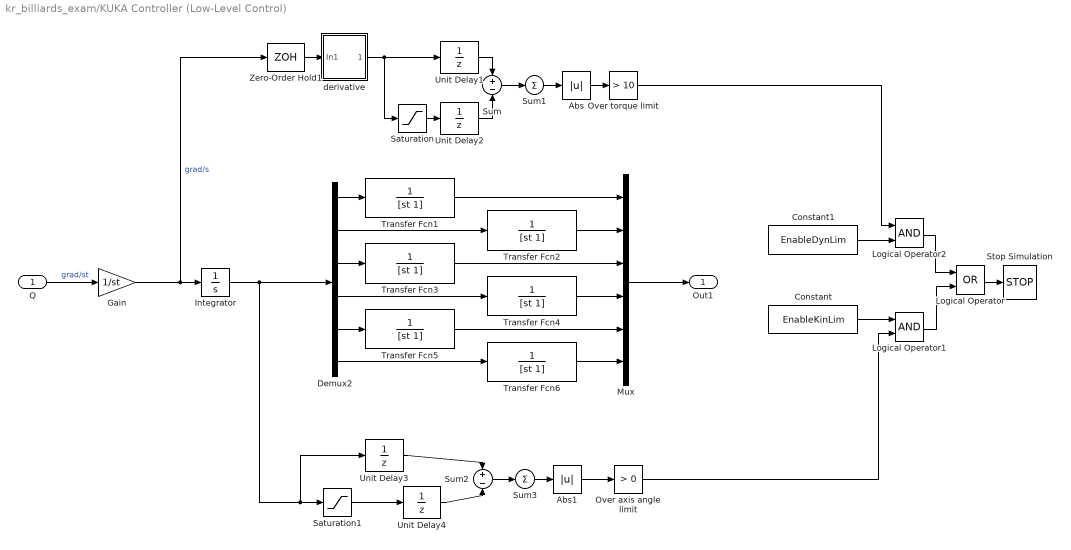
== system kr_billiards_exam/KUKA Controller (Low-Level Control) ==
  Q : Inport
  Abs : Abs
  Abs1 : Abs
  Constant : Constant  Value=EnableKinLim
  Constant1 : Constant  Value=EnableDynLim
  Demux2 : Demux  Outputs=6
  Gain : Gain  Gain=1/st
  Integrator : Integrator
  Logical Operator : Logic  Operator=OR  AllPortsSameDT=off  OutDataTypeStr=boolean
  Logical Operator1 : Logic  AllPortsSameDT=off  OutDataTypeStr=boolean
  Logical Operator2 : Logic  AllPortsSameDT=off  OutDataTypeStr=boolean
  Mux : Mux  Inputs=6
  Over axis angle limit : simulink/Logic and Bit Operations/Compare To Constant  relop=>  const=0  OutDataTypeStr=boolean
  Over torque limit : simulink/Logic and Bit Operations/Compare To Constant  relop=>  const=10  OutDataTypeStr=boolean
  Saturation : Saturate  UpperLimit=[acc1 acc2 acc3 acc4 acc5 acc6]  LowerLimit=-[acc1 acc2 acc3 acc4 acc5 acc6]
  Saturation1 : Saturate  UpperLimit=[max1 max2 max3 max4 max5 max6]  LowerLimit=[min1 min2 min3 min4 min5 min6]
  Stop Simulation : Stop
  Sum : Sum  Inputs=+|-
  Sum1 : Sum  Inputs=+
  Sum2 : Sum  Inputs=+|-
  Sum3 : Sum  Inputs=+
  Transfer Fcn{1..6} (6 alike) : TransferFcn  Denominator=[st 1]
  Unit Delay{1..4} (4 alike) : UnitDelay  SampleTime=st
  Zero-Order Hold1 : ZeroOrderHold  SampleTime=st
  derivative : Subsystem
  Out1 : Outport
  wires:
  Q/1 -> Gain/1  "grad/st"
  Transfer Fcn5/1 -> Mux/5
  Transfer Fcn3/1 -> Mux/3
  Demux2/3 -> Transfer Fcn3/1
  Demux2/5 -> Transfer Fcn5/1
  Demux2/1 -> Transfer Fcn1/1
  Transfer Fcn1/1 -> Mux/1
  Demux2/6 -> Transfer Fcn6/1
  Demux2/4 -> Transfer Fcn4/1
  Demux2/2 -> Transfer Fcn2/1
  Transfer Fcn6/1 -> Mux/6
  Transfer Fcn4/1 -> Mux/4
  Transfer Fcn2/1 -> Mux/2
  derivative/1(Out1) -> Saturation/1, Unit Delay1/1
  Mux/1 -> Out1/1
  Saturation/1 -> Unit Delay2/1
  Saturation1/1 -> Unit Delay4/1
  Unit Delay1/1 -> Sum/1
  Unit Delay2/1 -> Sum/2
  Sum/1 -> Sum1/1
  Over torque limit/1 -> Logical Operator2/1
  Sum1/1 -> Abs/1
  Abs/1 -> Over torque limit/1
  Unit Delay3/1 -> Sum2/1
  Unit Delay4/1 -> Sum2/2
  Sum2/1 -> Sum3/1
  Sum3/1 -> Abs1/1
  Abs1/1 -> Over axis angle limit/1
  Logical Operator1/1 -> Logical Operator/2
  Logical Operator/1 -> Stop Simulation/1
  Constant/1 -> Logical Operator1/1
  Over axis angle limit/1 -> Logical Operator1/2
  Logical Operator2/1 -> Logical Operator/1
  Constant1/1 -> Logical Operator2/2
  Integrator/1 -> Unit Delay3/1, Saturation1/1, Demux2/1
  Zero-Order Hold1/1 -> derivative/1(In1)
  Gain/1 -> Zero-Order Hold1/1, Integrator/1  "grad/s"
